simulink model "case1"  (R2019a)
settings: Solver=VariableStepAuto  StartTime=0.0  StopTime=250  RelTol=1e-3
values from neighbouring files (symbols this model uses):
  A = 33    [kalman_dynamic.m]
  a = 0.16    [kalman_dynamic.m]
libraries: R7014E_lib x2
settings Model: Creator=marbla-6  LastModifiedBy=marbla-6
settings SolverCC: ZeroCrossAlgorithm=Adaptive
settings DebuggingCC: IgnoredZcDiagnostic=none

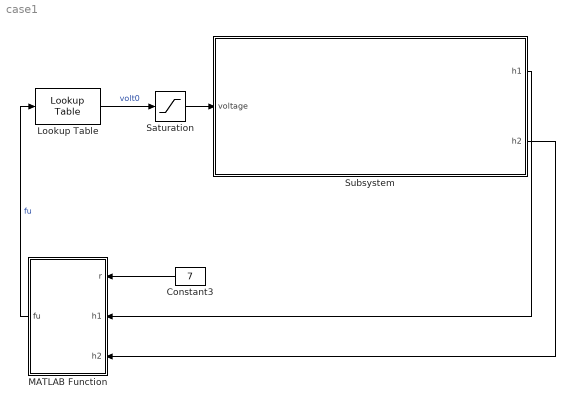
== system case1 ==
  Constant3 : Constant  Value=7
  Lookup Table : R7014E_lib/Lookup Table  x=[16.47,20.75,24.52,27.63,30.06,32.49,34.8,40.28,48.24,52.43]  y=[0.5,1,1.5,2,2.5,3,3.5,5,8,10]
  MATLAB Function : MATLAB Function  TreatAsAtomicUnit=on
  Saturation : Saturate  UpperLimit=10  LowerLimit=0
  Subsystem : Subsystem
  wires:
  Constant3/1 -> MATLAB Function/1(r)
  MATLAB Function/1(fu) -> Lookup Table/1  "fu"
  Lookup Table/1 -> Saturation/1  "volt0"
  Subsystem/1(h1) -> MATLAB Function/2(h1)
  Subsystem/2(h2) -> MATLAB Function/3(h2)
  Saturation/1 -> Subsystem/1(voltage)

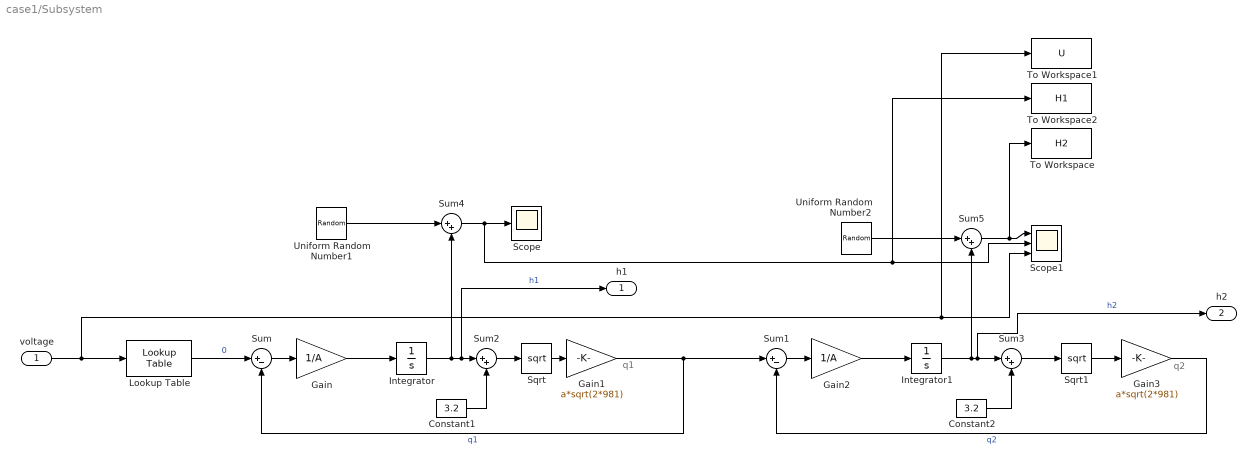
== system case1/Subsystem ==
  note: q1
  note: q2
  voltage : Inport
  Constant1 : Constant  Value=3.2
  Constant2 : Constant  Value=3.2
  Gain : Gain  Gain=1/A
  Gain1 : Gain  Gain=a*sqrt(2*981)
  Gain2 : Gain  Gain=1/A
  Gain3 : Gain  Gain=a*sqrt(2*981)
  Integrator : Integrator  LimitOutput=on  UpperSaturationLimit=15.5  LowerSaturationLimit=0
  Integrator1 : Integrator  LimitOutput=on  UpperSaturationLimit=15.5  LowerSaturationLimit=0
  Lookup Table : R7014E_lib/Lookup Table  x=[0.5,1,1.5,2,2.5,3,3.5,5,8,10]  y=[16.47,20.75,24.52,27.63,30.06,32.49,34.8,40.28,48.24,52.43]
  Scope : Scope
  Scope1 : Scope  NumInputPorts=3
  Sqrt : Sqrt  SaturateOnIntegerOverflow=on
  Sqrt1 : Sqrt  SaturateOnIntegerOverflow=on
  Sum : Sum  Inputs=|+-
  Sum1 : Sum  Inputs=|+-
  Sum{2..5} (4 alike) : Sum  Inputs=|++
  To Workspace : ToWorkspace  VariableName=H2  SaveFormat=Timeseries  SampleTime=-1
  To Workspace1 : ToWorkspace  VariableName=U  SaveFormat=Timeseries  SampleTime=-1
  To Workspace2 : ToWorkspace  VariableName=H1  SaveFormat=Timeseries  SampleTime=-1
  Uniform Random Number1 : UniformRandomNumber  Minimum=-0.1  Maximum=0.1  SampleTime=0.1
  Uniform Random Number2 : UniformRandomNumber  Minimum=-0.1  Maximum=0.1  SampleTime=0.1
  h1 : Outport
  h2 : Outport  Port=2
  wires:
  Lookup Table/1 -> Sum/1  "0"
  Sum3/1 -> Sqrt1/1
  Sum2/1 -> Sqrt/1
  Integrator1/1 -> h2/1, Sum3/1, Sum5/2  "h2"
  Gain1/1 -> Sum1/1, Sum/2  "q1"
  Gain2/1 -> Integrator1/1
  Integrator/1 -> h1/1, Sum2/1, Sum4/2  "h1"
  Constant2/1 -> Sum3/2
  Constant1/1 -> Sum2/2
  voltage/1 -> To Workspace1/1, Scope1/3, Lookup Table/1
  Sum5/1 -> Scope1/1, To Workspace/1
  Sum1/1 -> Gain2/1
  Sqrt1/1 -> Gain3/1
  Gain/1 -> Integrator/1
  Gain3/1 -> Sum1/2  "q2"
  Sqrt/1 -> Gain1/1
  Sum/1 -> Gain/1
  Sum4/1 -> To Workspace2/1, Scope1/2, Scope/1
  Uniform Random Number1/1 -> Sum4/1
  Uniform Random Number2/1 -> Sum5/1

== matlab function case1/MATLAB Function ==
  data: r input; h1 input; fu output; h2 input
function fu = fcn(r, h1, h2)

    % h1, h2 are including outlet height
    
    a = 0.16;
    A = 33;
    g = 982;
    h0 = 3.2;
    

    p1=-0.2;
    p2=-0.2;
    

    l_1 = -p1-p2;
    l_2 = p1*p2;
    
    L = [l_2 l_1];
    Lr = l_2;
    
    alpha = -(a^2/A^2)*g*sqrt((h1+h0)/(h2+h0));
    beta = (a/(2*A^2))*sqrt((2*g)/(h1+h0));
    h2_dot = (a/A)*sqrt(2*g)*(sqrt(h1+h0)-sqrt(h2+h0));
    
    x1 = h2;
    x2 = h2_dot;  
    x = [x1; x2];
    
  
    fu = (1/beta)*(-L*x+Lr*r-alpha);
    
end
